simulink model "TST01_circuitoRLC"  (R2023a)
settings: Solver=VariableStepAuto  StartTime=0.0  StopTime=10  RelTol=1e-3
settings Model: Creator=admin  LastModifiedBy=admin

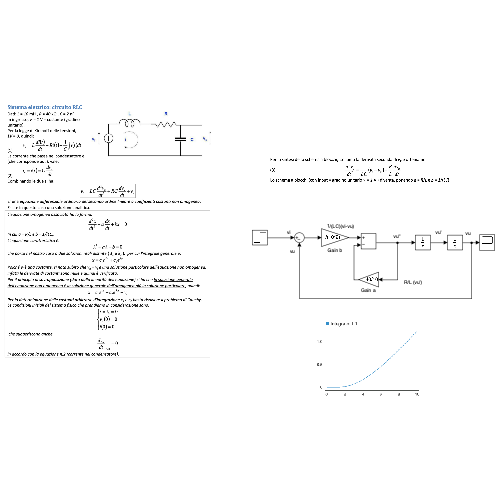
[thumbnail: Simulink's stored preview of the top-level diagram]
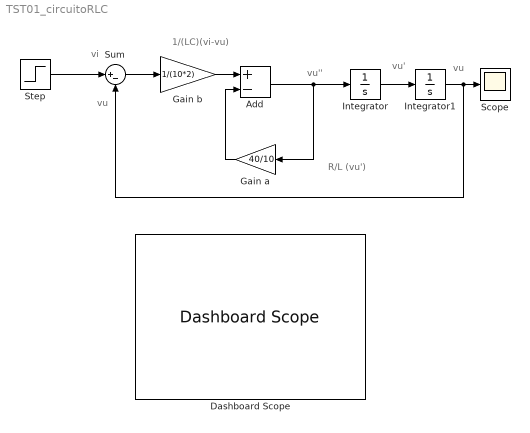
== system TST01_circuitoRLC ==
  note: R/L (vu')
  note: 1/(LC)(vi-vu)
  note: vu
  note: vu'
  note: vu''
  note: vu
  note: vi
  Add : Sum  Inputs=+-
  Dashboard Scope : DashboardScope
  Gain a : Gain  Gain=40/10
  Gain b : Gain  Gain=1/(10*2)
  Integrator : Integrator
  Integrator1 : Integrator
  Scope : Scope
  Step : Step  SampleTime=0
  Sum : Sum  Inputs=|+-
  wires:
  Step/1 -> Sum/1
  Sum/1 -> Gain b/1
  Gain b/1 -> Add/1
  Add/1 -> Integrator/1, Gain a/1
  Gain a/1 -> Add/2
  Integrator/1 -> Integrator1/1
  Integrator1/1 -> Sum/2, Scope/1
